simulink model "gm_newsimul"  (R2023a)
settings: Solver=FixedStepAuto  StartTime=0.0  StopTime=50e-6 - 1/2e9  RelTol=1e-3  EnableMultiTasking=on
undefined symbols (not defined in the file or in its folder): Add, Shift, yr_c
libraries: hdlsllib x3, dsphdlfiltering2 x1, dsphdlmathfun2 x1
settings Model: Creator=Windows User  LastModifiedBy=Windows User
settings OptimizationCC: BlockReduction=off  ConditionallyExecuteInputs=off  DefaultParameterBehavior=Inlined
settings DebuggingCC: AlgebraicLoopMsg=error  InheritedTsInSrcMsg=none  SingleTaskRateTransMsg=error
settings HardwareCC: ProdBitPerPointer=32  ProdBitPerSizeT=32  ProdBitPerPtrDiffT=32  ProdLargestAtomicFloat=None  ProdIntDivRoundTo=Undefined  ProdEndianess=Unspecified  ProdWordSize=32  ProdHWDeviceType=ASIC/FPGA->ASIC/FPGA  TargetBitPerPointer=64  TargetBitPerSizeT=64  TargetBitPerPtrDiffT=64  TargetLongLongMode=on  TargetIntDivRoundTo=Zero  TargetEndianess=LittleEndian  TargetWordSize=64  TargetHWDeviceType=Custom Processor->MATLAB Host Computer  ProdEqTarget=off

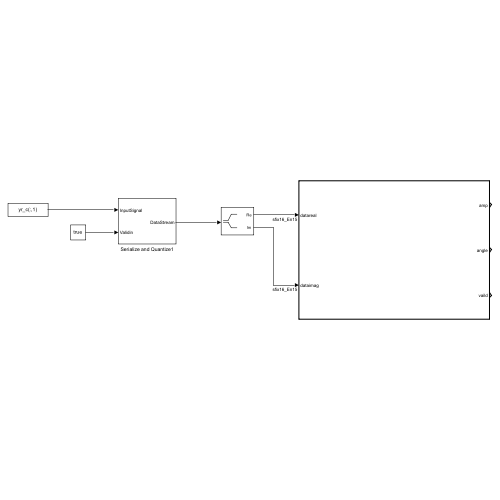
[thumbnail: Simulink's stored preview of the top-level diagram]
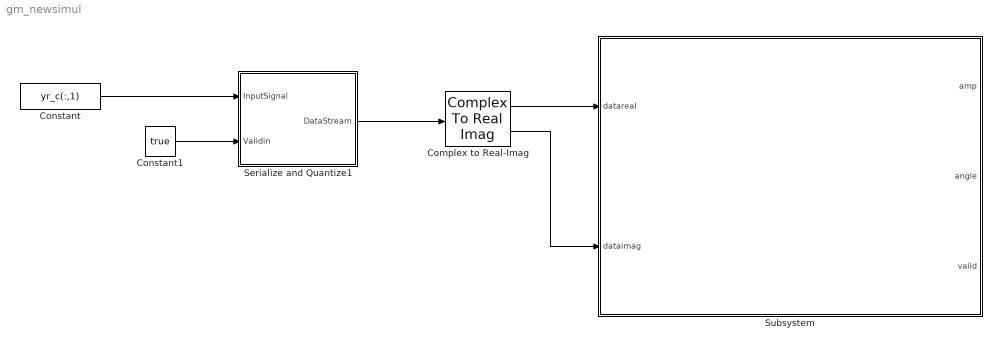
== system gm_newsimul ==
  Complex to Real-Imag : ComplexToRealImag
  Constant : Constant  Value=yr_c(:,1)  SampleTime=50e-6
  Constant1 : Constant  Value=true  OutDataTypeStr=boolean
  Serialize and Quantize1 : Subsystem
  Subsystem : Subsystem  TreatAsAtomicUnit=on
  wires:
  Constant/1 -> Serialize and Quantize1/1(InputSignal)
  Complex to Real-Imag/2 -> Subsystem/2(dataimag)
  Complex to Real-Imag/1 -> Subsystem/1(datareal)
  Serialize and Quantize1/1(DataStream) -> Complex to Real-Imag/1
  Constant1/1 -> Serialize and Quantize1/2(Validin)

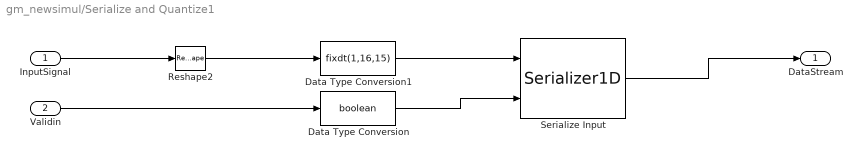
== system gm_newsimul/Serialize and Quantize1 ==
  InputSignal : Inport
  Validin : Inport  Port=2
  Data Type Conversion : DataTypeConversion  OutDataTypeStr=boolean  SaturateOnIntegerOverflow=off  RndMeth=Floor
  Data Type Conversion1 : DataTypeConversion  OutDataTypeStr=fixdt(1,16,15)  SaturateOnIntegerOverflow=off  RndMeth=Floor
  Reshape2 : Reshape  OutputDimensionality=Column vector (2-D)
  Serialize Input : hdlsllib/HDL Operations/Serializer1D  Ratio=100000  IdleCycles=0  validIn=on  startOut=off  validOut=off  inputDataDimensions=-1  inputSampleTime=-1  inputSignalType=auto
  DataStream : Outport
  wires:
  Data Type Conversion1/1 -> Serialize Input/1
  Reshape2/1 -> Data Type Conversion1/1
  Serialize Input/1 -> DataStream/1
  Data Type Conversion/1 -> Serialize Input/2
  Validin/1 -> Data Type Conversion/1
  InputSignal/1 -> Reshape2/1

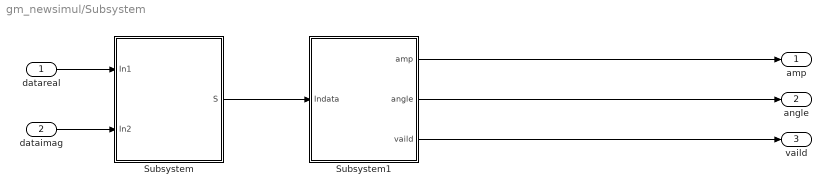
== system gm_newsimul/Subsystem ==
  datareal : Inport  OutDataTypeStr=fixdt(1, 16, 15)  PortDimensions=1  SampleTime=5e-10
  dataimag : Inport  Port=2  OutDataTypeStr=fixdt(1, 16, 15)  PortDimensions=1  SampleTime=5e-10
  Subsystem : Subsystem
  Subsystem1 : Subsystem
  amp : Outport  SampleTime=5e-10
  angle : Outport  Port=2  SampleTime=5e-10
  vaild : Outport  Port=3  SampleTime=5e-10
  wires:
  datareal/1 -> Subsystem/1(In1)
  dataimag/1 -> Subsystem/2(In2)
  Subsystem/1(S) -> Subsystem1/1(Indata)
  Subsystem1/1(amp) -> amp/1
  Subsystem1/2(angle) -> angle/1
  Subsystem1/3(vaild) -> vaild/1

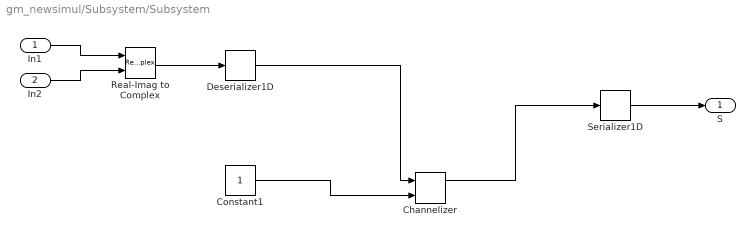
== system gm_newsimul/Subsystem/Subsystem ==
  In1 : Inport  OutDataTypeStr=fixdt(1, 16, 15)  PortDimensions=1  SampleTime=5e-10
  In2 : Inport  Port=2  OutDataTypeStr=fixdt(1, 16, 15)  PortDimensions=1  SampleTime=5e-10
  Channelizer : dsphdlfiltering2/Channelizer  FilterCoefficients=LowpassCoefficients  FilterStructure=Direct form transposed  NumFrequencyBands=FFTLength  ComplexMultiplication=Use 4 multipliers and 2 adders  Normalize=on  OutputSize=Same as input size  SimulateUsing=Code generation  roundingMode=Floor  overflowMode=off  CoefficientsDataTypeStr=Inherit: Same word length as input  FilterOutputDataTypeStr=fixdt(1,16,15)  ResetInputPort=off  StartOutputPort=off  EndOutputPort=off
  Constant1 : Constant  OutDataTypeStr=boolean  SampleTime=1.6e-08
  Deserializer1D : hdlsllib/HDL Operations/Deserializer1D  Ratio=32  IdleCycles=0  InitialCondition=0+0i  startIn=off  validIn=off  validOut=off  inputDataDimensions=1  inputSampleTime=5e-10  inputSignalType=complex
  Real-Imag to Complex : RealImagToComplex  ConstantPart="fi(0,1,16,15,\"hex\",\"0000\")"  SampleTime=5e-10
  Serializer1D : hdlsllib/HDL Operations/Serializer1D  Ratio=32  IdleCycles=0  validIn=off  startOut=off  validOut=off  inputDataDimensions=32  inputSampleTime=1.6e-08  inputSignalType=complex
  S : Outport  SampleTime=5e-10
  wires:
  In1/1 -> Real-Imag to Complex/1
  In2/1 -> Real-Imag to Complex/2
  Channelizer/1 -> Serializer1D/1
  Constant1/1 -> Channelizer/2
  Serializer1D/1 -> S/1
  Deserializer1D/1 -> Channelizer/1
  Real-Imag to Complex/1 -> Deserializer1D/1

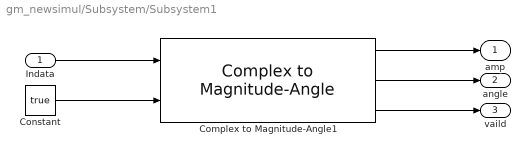
== system gm_newsimul/Subsystem/Subsystem1 ==
  Indata : Inport  OutDataTypeStr=fixdt(1, 16, 15)  PortDimensions=1  SampleTime=5e-10
      settings: SignalType=complex
  Complex to Magnitude-Angle1 : dsphdlmathfun2/Complex to Magnitude-Angle  NumIterationsSource=Property  NumIterations=15  OutputFormat=Magnitude and angle  AngleFormat=Radians  ScaleOutput=on  ScalingMethod=Shift-Add  SimulateUsing=Code generation
  Constant : Constant  Value=true  OutDataTypeStr=boolean  SampleTime=-1
  amp : Outport  SampleTime=5e-10
  angle : Outport  Port=2  SampleTime=5e-10
  vaild : Outport  Port=3  SampleTime=5e-10
  wires:
  Indata/1 -> Complex to Magnitude-Angle1/1
  Complex to Magnitude-Angle1/1 -> amp/1
  Complex to Magnitude-Angle1/2 -> angle/1
  Complex to Magnitude-Angle1/3 -> vaild/1
  Constant/1 -> Complex to Magnitude-Angle1/2
